simulink model "model"  (Simulink 7.1)
settings: Solver=FixedStepDiscrete  StartTime=0.0  StopTime=10.0  FixedStep=0.1  RelTol=1e-3
PreLoadFcn:
  | PolyModelTest
values from neighbouring files (symbols this model uses):
  A = y.A    [A_BLOM_MatMul.m]    (also in BLOM_EvalPolyBlock.m = A(any(C,1),:); BLOM_TranposeMat.m = Ain; BLOM_diagMat.m = Ain; CreateProblemCBs.m = [])
  C = y.C    [A_BLOM_MatMul.m]    (also in BLOM_EvalPolyBlock.m = C(:,any(C,1)); BLOM_TranposeMat.m = Cin(mat_idx(:),:); BLOM_diagMat.m = Cin(mat_idx(:),:))
undefined symbols (not defined in the file or in its folder): A2
libraries: MPCMdlLib x12, simulink x1
settings Model: Creator=vichik  LastModifiedBy=vichik

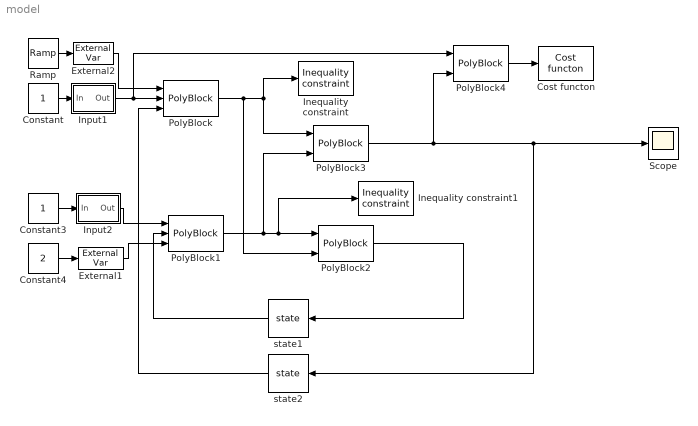
== system model ==
  Constant : Constant  OutDataType=sfix(16)  OutScaling=2^0
  Constant3 : Constant  OutDataType=sfix(16)  OutScaling=2^0
  Constant4 : Constant  Value=2  OutDataType=sfix(16)  OutScaling=2^0
  Cost functon : MPCMdlLib/Cost functon  Tag=OptCost
  External1 : MPCMdlLib/External Var  Tag=OptExternal  SystemSampleTime=-1
  External2 : MPCMdlLib/External Var  Tag=OptExternal  SystemSampleTime=-1
  Inequality constraint : MPCMdlLib/Inequality constraint  Tag=InequalBlock  CompareSign=> 0
  Inequality constraint1 : MPCMdlLib/Inequality constraint  Tag=InequalBlock  CompareSign=< 0
  Input1 : Subsystem  Tag=OptInput  AncestorBlock=MPCMdlLib/Input var  mask{step_ratio=1, data_name='fjglkdf'}
      mask prompts: step_ratio "Step ratio"
  Input2 : Subsystem  Tag=OptInput  AncestorBlock=MPCMdlLib/Input var  mask{step_ratio=2, data_name='gdhd'}
      mask prompts: step_ratio "Step ratio"
  PolyBlock : MPCMdlLib/PolyBlock  Tag=PolyBlock  A=A  C=C
  PolyBlock1 : MPCMdlLib/PolyBlock  Tag=PolyBlock  A=A  C=C
  PolyBlock2 : MPCMdlLib/PolyBlock  Tag=PolyBlock  A=A2  C=C
  PolyBlock3 : MPCMdlLib/PolyBlock  Tag=PolyBlock  A=A2  C=C
  PolyBlock4 : MPCMdlLib/PolyBlock  Tag=PolyBlock  A=A2  C=C
  Ramp : simulink/Sources/Ramp  SystemSampleTime=-1  slope=1  start=0  X0=0
  Scope : Scope
      settings: TimeRange=10
  state1 : MPCMdlLib/state  Tag=OptState  Orientation=left  SystemSampleTime=-1
  state2 : MPCMdlLib/state  Tag=OptState  Orientation=left  SystemSampleTime=-1
  wires:
  PolyBlock/1 -> PolyBlock3/1, Inequality constraint/1, PolyBlock2/2
  PolyBlock1/1 -> PolyBlock3/2, PolyBlock2/1, Inequality constraint1/1
  Constant3/1 -> Input2/1(In)
  Constant4/1 -> External1/1
  PolyBlock3/1 -> Scope/1, state2/1, PolyBlock4/2
  Ramp/1 -> External2/1
  Constant/1 -> Input1/1(In)
  PolyBlock2/1 -> state1/1
  state1/1 -> PolyBlock1/2
  state2/1 -> PolyBlock/3
  Input1/1(Out) -> PolyBlock/2, PolyBlock4/1
  Input2/1(Out) -> PolyBlock1/1
  External1/1 -> PolyBlock1/3
  External2/1 -> PolyBlock/1
  PolyBlock4/1 -> Cost functon/1

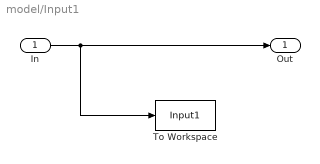
== system model/Input1 ==
  In : Inport  OutDataType=fixdt(1, 16)  OutScaling=2^0
  To Workspace : ToWorkspace  VariableName=Input1  SampleTime=-1  SaveFormat=Structure
      settings: InitFcn=set_param(getfullname(gcb),'VariableName',get_param(get_param(gcb,'parent'),'name'))
  Out : Outport  OutDataType=fixdt(1, 16)  OutScaling=2^0
  wires:
  In/1 -> To Workspace/1, Out/1

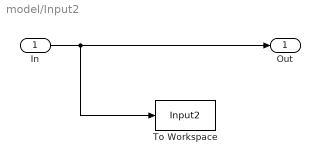
== system model/Input2 ==
  In : Inport  OutDataType=fixdt(1, 16)  OutScaling=2^0
  To Workspace : ToWorkspace  VariableName=Input2  SampleTime=-1  SaveFormat=Structure
      settings: InitFcn=set_param(getfullname(gcb),'VariableName',get_param(get_param(gcb,'parent'),'name'))
  Out : Outport  OutDataType=fixdt(1, 16)  OutScaling=2^0
  wires:
  In/1 -> To Workspace/1, Out/1
